simulink model "start_stop"  (R2021a)
settings: Solver=VariableStepAuto  StartTime=0.0  StopTime=10.0  RelTol=1e-3
libraries: simulink x4
settings Model: Creator=thyag  LastModifiedBy=thyag

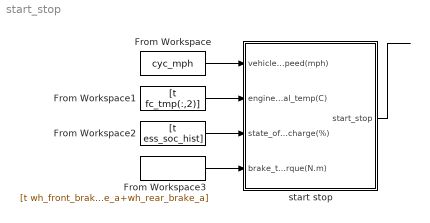
== system start_stop ==
  From Workspace : FromWorkspace  VariableName=cyc_mph
  From Workspace1 : FromWorkspace  VariableName=[t fc_tmp(:,2)]
  From Workspace2 : FromWorkspace  VariableName=[t ess_soc_hist]
  From Workspace3 : FromWorkspace  VariableName=[t wh_front_brake_a+wh_rear_brake_a]
  start stop : Subsystem  AncestorBlock=lib_controls/<vc> par/start stop
  wires:
  From Workspace3/1 -> start stop/4(brake_torque(N.m))
  start stop/1(start_stop) -> ?
  From Workspace1/1 -> start stop/2(engine_internal_temp(C))
  From Workspace2/1 -> start stop/3(state_of_charge(%))
  From Workspace/1 -> start stop/1(vehicle_speed(mph))

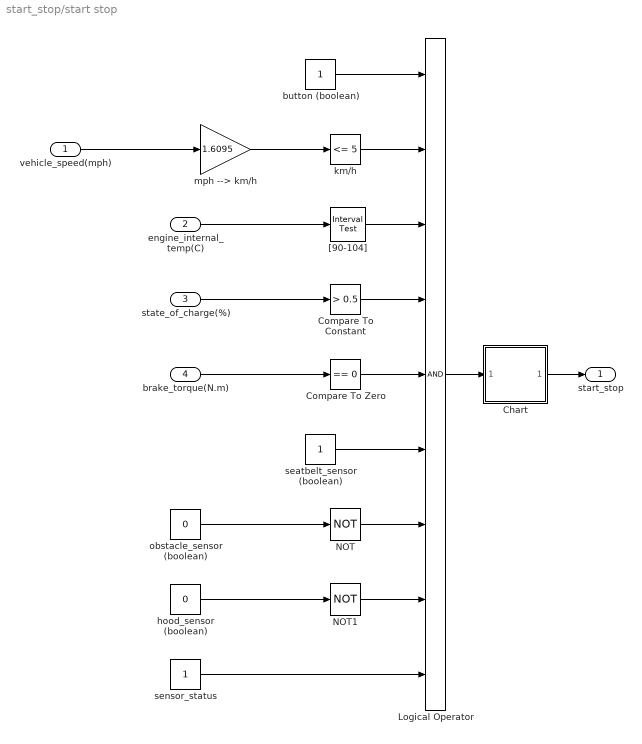
== system start_stop/start stop ==
  vehicle_speed(mph) : Inport
  engine_internal_temp(C) : Inport  Port=2
  state_of_charge(%) : Inport  Port=3
  brake_torque(N.m) : Inport  Port=4
  Chart : Stateflow chart  TreatAsAtomicUnit=on
  Compare To Constant : simulink/Logic and Bit Operations/Compare To Constant  relop=>  const=0.5  OutDataTypeStr=boolean
  Compare To Zero : simulink/Logic and Bit Operations/Compare To Zero  relop===  OutDataTypeStr=boolean
  Logical Operator : Logic  Inputs=9  AllPortsSameDT=off  OutDataTypeStr=boolean
  NOT : Logic  Operator=NOT  IconShape=distinctive  AllPortsSameDT=off  OutDataTypeStr=boolean
  NOT1 : Logic  Operator=NOT  IconShape=distinctive  AllPortsSameDT=off  OutDataTypeStr=boolean
  "[90-104]" : simulink/Logic and Bit Operations/Interval Test  IntervalClosedRight=on  uplimit=104  IntervalClosedLeft=on  lowlimit=90  OutDataTypeStr=boolean
  button (boolean) : Constant
  hood_sensor (boolean) : Constant  Value=0
  km/h : simulink/Logic and Bit Operations/Compare To Constant  relop=<=  const=5  OutDataTypeStr=boolean
  mph --> km/h : Gain  Gain=1.6095
  obstacle_sensor (boolean) : Constant  Value=0
  seatbelt_sensor (boolean) : Constant
  sensor_status : Constant
  start_stop : Outport
  wires:
  sensor_status/1 -> Logical Operator/9
  Logical Operator/1 -> Chart/1(condition)
  km/h/1 -> Logical Operator/2
  engine_internal_temp(C)/1 -> "[90-104]"/1
  Chart/1(engine) -> start_stop/1
  vehicle_speed(mph)/1 -> mph --> km/h/1
  state_of_charge(%)/1 -> Compare To Constant/1
  mph --> km/h/1 -> km/h/1
  Compare To Zero/1 -> Logical Operator/5
  brake_torque(N.m)/1 -> Compare To Zero/1
  seatbelt_sensor (boolean)/1 -> Logical Operator/6
  NOT/1 -> Logical Operator/7
  Compare To Constant/1 -> Logical Operator/4
  NOT1/1 -> Logical Operator/8
  "[90-104]"/1 -> Logical Operator/3
  hood_sensor (boolean)/1 -> NOT1/1
  obstacle_sensor (boolean)/1 -> NOT/1
  button (boolean)/1 -> Logical Operator/1

== stateflow chart start_stop/start stop/Chart ==
  state On
    entry:
    engine = 0;
  state Off
    entry:
    engine = 1;
  (default) -> On
  On -> Off : [condition == false]
  Off -> On : [condition == true]
  data: condition input; engine output
